simulink model "BANSHEE"  (Simulink 8.1)
settings: Solver=ode1  StartTime=0.0  StopTime=inf  FixedStep=Ts  MaxStep=1e-3  RelTol=1e-3
PostLoadFcn:
  | BANSHEE_init;
InitFcn:
  | BANSHEE_init;
undefined symbols (not defined in the file or in its folder): cable_spec, F1, F2, F3, fdesignblkfcn, Feeder1_lib, Feeder2_lib, Feeder3_lib, gcbh, generic_ethernet_cb, Left, relay_housing_lib, SM_UtilityService, SS_F1_RELAY_HOUSING, SS_F2_RELAY_HOUSING, SS_F3_RELAY_HOUSING, SS_Feeder1, SS_Feeder2, SS_Feeder3, Ts, type, utility_service_lib, V
libraries: breaker_lib x51, rtio_generic_modbus x43, relay_modbus_lib x42, cables_lib x34, artemis x24, transformer_lib x24, Load_lib x20, simulink x16, ssn_lib x16, rtlab x15, rtio_opalrt_common x15, PQFV_lib x8
(part 4 of 5)

== system BANSHEE/SM_UtilityService/HWCtrl_IOs ==
  note: When the system uses the simulated
      | Secondary Controller the digital I/O
      | should be disabled.
  note: Copyright (c) 2016 Massachusetts Institute of Technology
      | Permission is hereby granted, free of charge, to any person obtaining a copy of this software and associated documentation files (the "Software"), to deal
      | in the Software without restriction, including without limitation the rights to use, copy, modify, merge, publish, distribute, sublicense, and/or sell copies of the
      | Software, and to permit persons to whom the Software is furnished to do so, subject to the following conditions:
      |
      | THE SOFTWARE IS PROVIDED "AS IS", WITHOUT WARRANTY OF ANY KIND, EXPRESS OR IMPLIED, INCLUDING BUT NOT LIMITED TO THE
      | WARRANTIES OF MERCHANTABILITY, FITNESS FOR A PARTICULAR PURPOSE AND NONINFRINGEMENT. IN NO EVENT SHALL THE AUTHORS
      | OR COPYRIGHT HOLDERS BE LIABLE FOR ANY CLAIM, DAMAGES OR OTHER LIABILITY, WHETHER IN AN ACTION OF CONTRACT, TORT OR
      | OTHERWISE, ARISING FROM, OUT OF OR IN CONNECTION WITH THE SOFTWARE OR THE USE OR OTHER DEALINGS IN THE SOFTWARE
  ScaledSignals : Inport
  Bus Creator : BusCreator
  Bus Creator1 : BusCreator  Inputs=5
  Bus Creator2 : BusCreator  Inputs=5
  Bus Creator3 : BusCreator  Inputs=2
  Bus Selector1 : BusSelector  OutputSignals=MCB_CB_Status
  Bus Selector2 : BusSelector  OutputSignals=scaled_gcb_voltage,scaled_gcb_current,scaled_mcb_voltage,scaled_mcb_current,scaled_speed
  Bus Selector3 : BusSelector  OutputSignals=NGCHP_ScaledSignals,Diesel_ScaledSignals
  Bus Selector4 : BusSelector  OutputSignals=scaled_gcb_voltage,scaled_gcb_current,scaled_mcb_voltage,scaled_mcb_current,scaled_speed
  Bus Selector5 : BusSelector  OutputSignals=MCB_CB_Status
  Demux1 : Demux  Outputs=16
  GR1 B AIN (CH00-15) : Subsystem
  Memory1 : Memory
  OpCtrl : rtio_opalrt_common/OpCtrl  CtrlName='OpCtrl'  boardid=0  BitstreamFilename=VC707_2-EX-0001-2_3_2_20-48AIO16DIO16DIOSel-02-01.bin  numconfig=-1  mode=Master  externalClock=off  decimRtsi=0  calibIO=off  SampleTime=0  loadinport=-1  BoardType=VC707  SecondaryPresent=off  sync_type=Audio
  Woodward Inputs : Subsystem
  Woodward Outputs - Diesel - Gen2 : Subsystem
  Woodward Outputs - NGCHP - Gen1 : Subsystem
  WoodwardBias : Outport
  wires:
  Bus Creator/1 -> [WoodwardBias]
  Memory1/1 -> WoodwardBias/1
  Bus Selector1/1 -> Woodward Outputs - NGCHP - Gen1/1(Gen1 MCB Status)  "<MCB_CB_Status>"
  [NGCHP_ScaledSignals] -> Bus Selector1/1
  [WoodwardBias] -> Woodward Outputs - NGCHP - Gen1/2(WoodwardBias)
  Woodward Outputs - NGCHP - Gen1/5(Gen1 MCB) -> Bus Creator2/5  "MCB_Ctrl"
  Woodward Outputs - Diesel - Gen2/1(Digital Inputs) -> Bus Creator1/1  "DIN"
  Woodward Outputs - NGCHP - Gen1/4(Gen1 GCB) -> Bus Creator2/4  "GCB_Crtl"
  Woodward Outputs - NGCHP - Gen1/3(Gen1 Fuel Enable) -> Bus Creator2/3  "FuelEnable"
  Woodward Outputs - NGCHP - Gen1/2(Gen1 Gov and AVR) -> Bus Creator2/2  "Gov_and_AVR"
  Woodward Outputs - NGCHP - Gen1/1(Digital Inputs) -> Bus Creator2/1  "DIN"
  Bus Creator2/1 -> Bus Creator3/1  "NGCHP_Gen1"
  Bus Creator3/1 -> Memory1/1
  Bus Creator1/1 -> Bus Creator3/2  "Diesel_Gen2"
  Woodward Outputs - Diesel - Gen2/5(Gen2 MCB) -> Bus Creator1/5  "MCB_Ctrl"
  Woodward Outputs - Diesel - Gen2/4(Gen2 GCB) -> Bus Creator1/4  "GCB_Crtl"
  Woodward Outputs - Diesel - Gen2/3(Gen2 Fuel Enable) -> Bus Creator1/3  "FuelEnable"
  Woodward Outputs - Diesel - Gen2/2(Gen2 Gov and AVR) -> Bus Creator1/2  "Gov_and_AVR"
  [Diesel_ScaledSignals] -> Bus Selector5/1
  [WoodwardBias] -> Woodward Outputs - Diesel - Gen2/2(WoodwardBias)
  Bus Selector5/1 -> Woodward Outputs - Diesel - Gen2/1(Gen2 MCB Status)  "<MCB_CB_Status>"
  Demux1/4 -> Bus Creator/4  "gen2_AVR_bias"
  Demux1/3 -> Bus Creator/3  "gen2_GOV_bias"
  Demux1/2 -> Bus Creator/2  "gen1_AVR_bias"
  Demux1/1 -> Bus Creator/1  "gen1_GOV_bias"
  GR1 B AIN (CH00-15)/1(Out1) -> Demux1/1
  Bus Selector4/5 -> Woodward Inputs/10(MPU2_speed)  "<scaled_speed>"
  Bus Selector4/4 -> Woodward Inputs/9(Mains2_Current)  "<scaled_mcb_current>"
  Bus Selector4/3 -> Woodward Inputs/8(Mains2_Voltage)  "<scaled_mcb_voltage>"
  Bus Selector4/2 -> Woodward Inputs/7(Generator2_Current)  "<scaled_gcb_current>"
  Bus Selector4/1 -> Woodward Inputs/6(Generator2_Voltage)  "<scaled_gcb_voltage>"
  [Diesel_ScaledSignals] -> Bus Selector4/1
  Bus Selector2/1 -> Woodward Inputs/1(Generator1_Voltage)  "<scaled_gcb_voltage>"
  Bus Selector2/2 -> Woodward Inputs/2(Generator1_Current)  "<scaled_gcb_current>"
  Bus Selector2/3 -> Woodward Inputs/3(Mains1_Voltage)  "<scaled_mcb_voltage>"
  Bus Selector2/4 -> Woodward Inputs/4(Mains1_Current)  "<scaled_mcb_current>"
  Bus Selector2/5 -> Woodward Inputs/5(MPU1_speed)  "<scaled_speed>"
  [NGCHP_ScaledSignals] -> Bus Selector2/1
  Bus Selector3/2 -> [Diesel_ScaledSignals]  "<Diesel_ScaledSignals>"
  Bus Selector3/1 -> [NGCHP_ScaledSignals]  "<NGCHP_ScaledSignals>"
  ScaledSignals/1 -> Bus Selector3/1

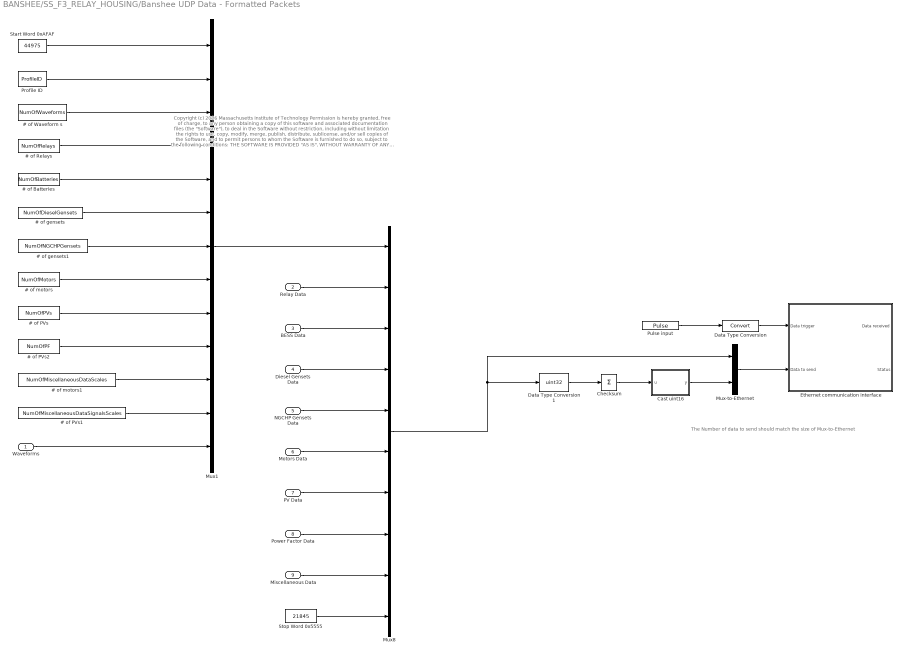
== system BANSHEE/SS_F3_RELAY_HOUSING/Banshee UDP Data - Formatted Packets ==
  note: The Number of data to send should match the size of Mux-to-Ethernet
  note: Copyright (c) 2016 Massachusetts Institute of Technology
      | Permission is hereby granted, free of charge, to any person obtaining a copy of this software and associated documentation files (the "Software"), to deal
      | in the Software without restriction, including without limitation the rights to use, copy, modify, merge, publish, distribute, sublicense, and/or sell copies of the
      | Software, and to permit persons to whom the Software is furnished to do so, subject to the following conditions:
      |
      | THE SOFTWARE IS PROVIDED "AS IS", WITHOUT WARRANTY OF ANY KIND, EXPRESS OR IMPLIED, INCLUDING BUT NOT LIMITED TO THE
      | WARRANTIES OF MERCHANTABILITY, FITNESS FOR A PARTICULAR PURPOSE AND NONINFRINGEMENT. IN NO EVENT SHALL THE AUTHORS
      | OR COPYRIGHT HOLDERS BE LIABLE FOR ANY CLAIM, DAMAGES OR OTHER LIABILITY, WHETHER IN AN ACTION OF CONTRACT, TORT OR
      | OTHERWISE, ARISING FROM, OUT OF OR IN CONNECTION WITH THE SOFTWARE OR THE USE OR OTHER DEALINGS IN THE SOFTWARE
  Waveforms : Inport  PortDimensions=3
  Relay Data : Inport  Port=2
  BESS Data : Inport  Port=3
  Diesel Gensets Data : Inport  Port=4
  NGCHP Gensets Data : Inport  Port=5
  Motors Data : Inport  Port=6
  PV Data : Inport  Port=7
  Power Factor Data : Inport  Port=8
  Miscellaneous Data : Inport  Port=9
  " # of motors" : Constant  Value=NumOfMotors  OutDataTypeStr=double
  " # of motors1" : Constant  Value=NumOfMiscellaneousDataScales  OutDataTypeStr=double
  # of Batteries : Constant  Value=NumOfBatteries  OutDataTypeStr=double
  # of PVs : Constant  Value=NumOfPVs  OutDataTypeStr=double
  # of PVs1 : Constant  Value=NumOfMiscellaneousDataSignalsScales  OutDataTypeStr=double
  # of PVs2 : Constant  Value=NumOfPF  OutDataTypeStr=double
  # of Relays : Constant  Value=NumOfRelays  OutDataTypeStr=double
  # of Waveform s : Constant  Value=NumOfWaveforms  OutDataTypeStr=double
  # of gensets : Constant  Value=NumOfDieselGensets  OutDataTypeStr=double
  # of gensets1 : Constant  Value=NumOfNGCHPGensets  OutDataTypeStr=double
  Cast uint16 : MATLAB Function  TreatAsAtomicUnit=on
  Checksum : Sum  Inputs=+
  Data Type Conversion : DataTypeConversion
  Data Type Conversion1 : DataTypeConversion  OutDataTypeStr=uint32  ConvertRealWorld=Stored Integer (SI)  RndMeth=Nearest
  Ethernet communication interface : Subsystem  mask(AsyncEthernet){ctrl_id=1, nbr_to_remote_endpoint=295, type_to_remote_endpoint=INT16, offset_to_remote_endpoint=0, swap_tx=off, nbr_from_remote_endpoint=4, type_from_remote_endpoint=UINT16, offset_from_remote_endpoint=0, swap_rx=off, exe_name='AsyncEthernet', nic_name='eth0', protocol=UDP, tcp_mode=Server, port=7200, remote_ip='255.255.255.255'}
      mask prompts: ctrl_id "Controller ID"; nbr_to_remote_endpoint "Number of data to send"; type_to_remote_endpoint "Type of data to send"; offset_to_remote_endpoint "Byte offset of transmission buffer"; swap_tx "Swap data endianness before transmission"; nbr_from_remote_endpoint "Number of data expected to be received"; type_from_remote_endpoint "Type of data expected to be received"; offset_from_remote_endpoint "Byte offset of reception buffer"; swap_rx "Swap data endianness after reception"; exe_name "Executable name"; nic_name "Network interface name"; tcp_mode "TCP mode"; port "Port number"; remote_ip "Remote IP address"
      mask help: This block is used as a communication interface to send data to a remote dedevice and receive data from it.
      mask Help: eval('rtlab_io_help(''Generic/Ethernet/Ethernet_interface.htm'');');
      mask Callback ctrl_id:
      | var = get_param(gcb,'ctrl_id');
      | set_param([gcb '/AsyncEthernetCtrl'],'ctrl_id',var)
      mask Callback nbr_to_remote_endpoint:
      | var = get_param(gcb,'nbr_to_remote_endpoint');
      | set_param([gcb '/AsyncEthernetCtrl'],'nbr_to_remote_endpoint',var)
      mask TypeOptions type_to_remote_endpoint: UINT8 | INT8 | UINT16 | INT16 | UINT32 | INT32 | FLOAT | DOUBLE
      mask Callback type_to_remote_endpoint:
      | var = get_param(gcb,'type_to_remote_endpoint');
      | set_param([gcb '/AsyncEthernetCtrl'],'type_to_remote_endpoint',var)
      mask Callback offset_to_remote_endpoint:
      | var = get_param(gcb,'offset_to_remote_endpoint');
      | set_param([gcb '/AsyncEthernetCtrl'],'offset_to_remote_endpoint',var)
      mask Callback swap_tx:
      | var = get_param(gcb,'swap_tx');
      | set_param([gcb '/AsyncEthernetCtrl'],'swap_tx',var)
      mask Callback nbr_from_remote_endpoint:
      | var = get_param(gcb,'nbr_from_remote_endpoint');
      | set_param([gcb '/AsyncEthernetCtrl'],'nbr_from_remote_endpoint',var)
      mask TypeOptions type_from_remote_endpoint: UINT8 | INT8 | UINT16 | INT16 | UINT32 | INT32 | FLOAT | DOUBLE
      mask Callback type_from_remote_endpoint:
      | var = get_param(gcb,'type_from_remote_endpoint');
      | set_param([gcb '/AsyncEthernetCtrl'],'type_from_remote_endpoint',var)
      mask Callback offset_from_remote_endpoint:
      | var = get_param(gcb,'offset_from_remote_endpoint');
      | set_param([gcb '/AsyncEthernetCtrl'],'offset_from_remote_endpoint',var)
      mask Callback swap_rx:
      | var = get_param(gcb,'swap_rx');
      | set_param([gcb '/AsyncEthernetCtrl'],'swap_rx',var)
      mask Callback exe_name:
      | str = get_param(gcb,'exe_name');
      | 
      | if exist('str','var')
      |     str = eval(str);
      | end
      | 
      | set_param([gcb '/AsyncEthernetCtrl'],'exe_name',str)
      mask Callback nic_name:
      | str = get_param(gcb,'nic_name');
      | 
      | if exist('str','var')
      |     str = eval(str);
      | end
      | 
      | set_param([gcb '/AsyncEthernetCtrl'],'nic_name',str)
      mask TypeOptions protocol: UDP | TCP
      mask Callback protocol: generic_ethernet_cb('protocol')
      mask TypeOptions tcp_mode: Client | Server
      mask Callback tcp_mode: generic_ethernet_cb('tcp_mode')
      mask Callback port:
      | var = get_param(gcb,'port');
      | set_param([gcb '/AsyncEthernetCtrl'],'port',var)
      mask Callback remote_ip:
      | str = get_param(gcb,'remote_ip');
      | 
      | if exist('str','var')
      |     str = eval(str);
      | end
      | 
      | set_param([gcb '/AsyncEthernetCtrl'],'remote_ip',str)
  Mux-to-Ethernet : Mux  Inputs=2
  Mux1 : Mux  Inputs=13
  Mux8 : Mux  Inputs=10
  Profile ID : Constant  Value=ProfileID  OutDataTypeStr=double
  Pulse input : DiscretePulseGenerator  PulseType=Time based  Period=1/5
  Start Word 0xAFAF : Constant  Value=44975  OutDataTypeStr=double
  Stop Word 0x5555 : Constant  Value=21845  OutDataTypeStr=double
  wires:
  # of Waveform s/1 -> Mux1/3
  Profile ID/1 -> Mux1/2
  Start Word 0xAFAF/1 -> Mux1/1
  Pulse input/1 -> Data Type Conversion/1
  Data Type Conversion/1 -> Ethernet communication interface/1(Data trigger)
  Mux1/1 -> Mux8/1
  Checksum/1 -> Cast uint16/1(u)
  Cast uint16/1(y) -> Mux-to-Ethernet/2
  Mux-to-Ethernet/1 -> Ethernet communication interface/2(Data to send)
  Data Type Conversion1/1 -> Checksum/1
  Waveforms/1 -> Mux1/13
  # of gensets/1 -> Mux1/6
  # of Batteries/1 -> Mux1/5
  # of Relays/1 -> Mux1/4
  BESS Data/1 -> Mux8/3
  Diesel Gensets Data/1 -> Mux8/4
  Relay Data/1 -> Mux8/2
  Mux8/1 -> Mux-to-Ethernet/1, Data Type Conversion1/1
  # of gensets1/1 -> Mux1/7
  " # of motors"/1 -> Mux1/8
  # of PVs/1 -> Mux1/9
  # of PVs2/1 -> Mux1/10
  " # of motors1"/1 -> Mux1/11
  # of PVs1/1 -> Mux1/12
  Stop Word 0x5555/1 -> Mux8/10
  NGCHP Gensets Data/1 -> Mux8/5
  Miscellaneous Data/1 -> Mux8/9
  Power Factor Data/1 -> Mux8/8
  PV Data/1 -> Mux8/7
  Motors Data/1 -> Mux8/6

== system BANSHEE/SS_F3_RELAY_HOUSING/SEL751-UDP ==
  note: Order of signals:
      | F3_PCC
      | F2_PCC
      | F1_PCC
      | F3_GCB (NG/CHP)
      | F1_GCB (DIESEL)
  note: % Copyright (c) 2016 Massachusetts Institute of Technology
      | % Permission is hereby granted, free of charge, to any person obtaining a copy of this
      | % software and associated documentation files (the "Software"), to deal in the Software
      | % without restriction, including without limitation the rights to use, copy, modify,
      | % merge, publish, distribute, sublicense, and/or sell copies of the Software, and to
      | % permit persons to whom the Software is furnished to do so, subject to the following
      | % conditions:
      | %
      | %
      | % The above copyright notice and this permission notice shall be included in
      | % all copies or substantial portions of the Software.
      | %
      | % THE SOFTWARE IS PROVIDED "AS IS", WITHOUT WARRANTY OF ANY KIND, EXPRESS OR IMPLIED,
      | % INCLUDING BUT NOT LIMITED TO THE WARRANTIES OF MERCHANTABILITY, FITNESS FOR A
      | % PARTICULAR PURPOSE AND NONINFRINGEMENT. IN NO EVENT SHALL THE AUTHORS OR COPYRIGHT
      | % HOLDERS BE LIABLE FOR ANY CLAIM, DAMAGES OR OTHER LIABILITY, WHETHER IN AN ACTION
      | % OF CONTRACT, TORT OR OTHERWISE, ARISING FROM, OUT OF OR IN CONNECTION WITH THE
      | % SOFTWARE OR THE USE OR OTHER DEALINGS IN THE SOFTWARE.
      | %
      | %
      | %%
  F3_MS : Inport
  F2_MS : Inport  Port=2
  F1_MS : Inport  Port=3
  Bus Creator : BusCreator  Inputs=5
  Bus Selector : BusSelector  OutputSignals=CB_DATA.F3_PCC
  Bus Selector3 : BusSelector  OutputSignals=CB_DATA.F2_PCC
  Bus Selector5 : BusSelector  OutputSignals=CB_DATA.F1_PCC
  PQFV : PQFV_lib/PQFV  VRMSLL=13800
  PQFV1 : PQFV_lib/PQFV  VRMSLL=13800
  PQFV2 : PQFV_lib/PQFV  VRMSLL=13800
  PQVF_out : Outport
  wires:
  Bus Selector/1 -> PQFV/1  "<F3_PCC>"
  Bus Selector3/1 -> PQFV1/1  "<F2_PCC>"
  F2_MS/1 -> Bus Selector3/1
  Bus Selector5/1 -> PQFV2/1  "<F1_PCC>"
  PQFV1/1 -> Bus Creator/2  "F2_PCC"
  PQFV/1 -> Bus Creator/1  "F3_PCC"
  PQFV2/1 -> Bus Creator/3  "F1_PCC"
  F3_MS/1 -> Bus Creator/4, Bus Selector/1  "F3_MS"
  F1_MS/1 -> Bus Creator/5, Bus Selector5/1  "F1_MS"
  Bus Creator/1 -> PQVF_out/1

== system BANSHEE/SS_Feeder3/HWController_3.5MVA_NGCHP ==
  note: Copyright (c) 2016 Massachusetts Institute of Technology
      | Permission is hereby granted, free of charge, to any person obtaining a copy of this software and associated documentation files (the "Software"), to deal
      | in the Software without restriction, including without limitation the rights to use, copy, modify, merge, publish, distribute, sublicense, and/or sell copies of the
      | Software, and to permit persons to whom the Software is furnished to do so, subject to the following conditions:
      |
      | THE SOFTWARE IS PROVIDED "AS IS", WITHOUT WARRANTY OF ANY KIND, EXPRESS OR IMPLIED, INCLUDING BUT NOT LIMITED TO THE
      | WARRANTIES OF MERCHANTABILITY, FITNESS FOR A PARTICULAR PURPOSE AND NONINFRINGEMENT. IN NO EVENT SHALL THE AUTHORS
      | OR COPYRIGHT HOLDERS BE LIABLE FOR ANY CLAIM, DAMAGES OR OTHER LIABILITY, WHETHER IN AN ACTION OF CONTRACT, TORT OR
      | OTHERWISE, ARISING FROM, OUT OF OR IN CONNECTION WITH THE SOFTWARE OR THE USE OR OTHER DEALINGS IN THE SOFTWARE
  In1 : Inport
  In2 : Inport  Port=2
  HWControllerBias : Inport  Port=3
  Bus Creator2 : BusCreator  Inputs=6
  Bus Selector6 : BusSelector  OutputSignals=Heat Recovered; MBtu/hr
  Bus Selector7 : BusSelector  OutputSignals=TempActual,HeatFromBoiler MBtu/hr,CHPHeatContribution MBtu/hr,Thermal data.Heat Recovered; MBtu/hr,Thermal data.CO2 lbm/hr
  CHPThermalModel : CHP_Model_lib/CHPThermalModel  SIM_HIL=SIM_HIL
  Demux : Demux  Outputs=2
  HWController_NG_Generator : HWController_NGCHP_Genset_3p5MVA_lib/HWController_NG_Generator
  Modbus device : rtio_generic_modbus/Modbus device  conf_name=CHP_slave_cfg.opal  conf_name_mask=CHP_slave_cfg.xls  sample_time=Ts
  Mux1 : Mux  Inputs=5
  A : PMIOPort  Tag=A  Port=1  Side=Right
      settings: AttributesFormatString=A
  B : PMIOPort  Port=2  Side=Right
  C : PMIOPort  Port=3  Side=Right
  Out1 : Outport
  Generator Data : Outport  Port=2
  GCB Control : Outport  Port=3
  wires:
  In2/1 -> CHPThermalModel/5  "CHP_SIM_Cmds"
  Bus Creator2/1 -> Bus Selector7/1, Out1/1  "CHPData"
  Bus Selector6/1 -> CHPThermalModel/1  "<Heat Recovered; MBtu/hr>"
  HWController_NG_Generator/2 -> GCB Control/1
  HWController_NG_Generator/1 -> Generator Data/1
  Modbus device/2 -> Demux/1
  [HeatRec_MBtuhr] -> Bus Selector6/1, Bus Creator2/2  "Thermal data"
  CHPThermalModel/3 -> Bus Creator2/4
  Demux/1 -> CHPThermalModel/3
  Mux1/1 -> Modbus device/4
  In1/1 -> CHPThermalModel/2
  Bus Selector7/1 -> Mux1/1  "<TempActual>"
  Bus Selector7/4 -> Mux1/4  "<Heat Recovered; MBtu/hr>"
  Bus Selector7/5 -> Mux1/5  "<CO2 lbm/hr>"
  Bus Selector7/2 -> Mux1/2  "<HeatFromBoiler MBtu/hr>"
  CHPThermalModel/2 -> Bus Creator2/3
  Demux/2 -> CHPThermalModel/4
  CHPThermalModel/1 -> Bus Creator2/1  "TempActual"
  Bus Selector7/3 -> Mux1/3  "<CHPHeatContribution MBtu/hr>"
  HWController_NG_Generator/3 -> [HeatRec_MBtuhr]  "Thermal data"
  HWControllerBias/1 -> HWController_NG_Generator/1
  CHPThermalModel/4 -> Bus Creator2/5
  CHPThermalModel/5 -> Bus Creator2/6
  connections:
  HWController_NG_Generator/RConn1 -- A/RConn1
  HWController_NG_Generator/RConn2 -- B/RConn1
  HWController_NG_Generator/RConn3 -- C/RConn1

== system BANSHEE/SC_ctrl/Overall/currents ==
  F1 : Inport
  F2 : Inport  Port=2
  F3 : Inport  Port=3
  1ph_rms1 : Subsystem
  1ph_rms10 : Subsystem
  1ph_rms11 : Subsystem
  1ph_rms12 : Subsystem
  1ph_rms13 : Subsystem
  1ph_rms14 : Subsystem
  1ph_rms15 : Subsystem
  1ph_rms2 : Subsystem
  1ph_rms3 : Subsystem
  1ph_rms4 : Subsystem
  1ph_rms5 : Subsystem
  1ph_rms6 : Subsystem
  1ph_rms7 : Subsystem
  1ph_rms8 : Subsystem
  1ph_rms9 : Subsystem
  Bus Selector : BusSelector  OutputSignals=F1_CB_1.m.Iabc,F1_CB_2.m.Iabc,F1_CB_3.m.Iabc,F1_CB_6.m.Iabc,F1_CB_10.m.Iabc
  Bus Selector1 : BusSelector  OutputSignals=F2_CB_1.m.Iabc,F2_CB_2.m.Iabc,F2_CB_3.m.Iabc,F2_CB_7.m.Iabc,F2_CB_14.m.Iabc,F2_CB_15.m.Iabc
  Bus Selector2 : BusSelector  OutputSignals=F3_CB_1.m.Iabc,F3_CB_2.m.Iabc,F3_CB_3.m.Iabc,F3_CB_4.m.Iabc
  Mux : Mux  Inputs=5
  Mux1 : Mux  Inputs=6
  Mux2 : Mux
  RMS_Calculator : Subsystem
  RMS_Calculator1 : Subsystem
  RMS_Calculator2 : Subsystem
  oF1 : Outport
  oF2 : Outport  Port=2
  oF3 : Outport  Port=3
  wires:
  Mux/1 -> RMS_Calculator/1(Signal)  "F1"
  Mux1/1 -> RMS_Calculator1/1(Signal)  "F2"
  Mux2/1 -> RMS_Calculator2/1(Signal)  "F3"
  Bus Selector/5 -> 1ph_rms3/1(i)  "<Iabc>"
  Bus Selector/4 -> 1ph_rms4/1(i)  "<Iabc>"
  Bus Selector/3 -> 1ph_rms2/1(i)  "<Iabc>"
  Bus Selector/2 -> 1ph_rms1/1(i)  "<Iabc>"
  Bus Selector/1 -> 1ph_rms6/1(i)  "<Iabc>"
  Bus Selector1/4 -> 1ph_rms9/1(i)  "<Iabc>"
  Bus Selector1/5 -> 1ph_rms13/1(i)  "<Iabc>"
  Bus Selector1/3 -> 1ph_rms8/1(i)  "<Iabc>"
  Bus Selector1/6 -> 1ph_rms10/1(i)  "<Iabc>"
  Bus Selector1/2 -> 1ph_rms7/1(i)  "<Iabc>"
  Bus Selector1/1 -> 1ph_rms5/1(i)  "<Iabc>"
  Bus Selector2/4 -> 1ph_rms15/1(i)  "<Iabc>"
  Bus Selector2/2 -> 1ph_rms12/1(i)  "<Iabc>"
  Bus Selector2/3 -> 1ph_rms11/1(i)  "<Iabc>"
  Bus Selector2/1 -> 1ph_rms14/1(i)  "<Iabc>"
  1ph_rms6/1(o) -> Mux/1
  1ph_rms1/1(o) -> Mux/2
  1ph_rms2/1(o) -> Mux/3
  1ph_rms3/1(o) -> Mux/5
  1ph_rms4/1(o) -> Mux/4
  1ph_rms5/1(o) -> Mux1/1
  1ph_rms7/1(o) -> Mux1/2
  1ph_rms8/1(o) -> Mux1/3
  1ph_rms9/1(o) -> Mux1/4
  1ph_rms14/1(o) -> Mux2/1
  1ph_rms13/1(o) -> Mux1/5
  1ph_rms10/1(o) -> Mux1/6
  1ph_rms12/1(o) -> Mux2/2
  1ph_rms11/1(o) -> Mux2/3
  1ph_rms15/1(o) -> Mux2/4
  RMS_Calculator/1(RMS_Signal) -> oF1/1
  RMS_Calculator1/1(RMS_Signal) -> oF2/1
  RMS_Calculator2/1(RMS_Signal) -> oF3/1
  F1/1 -> Bus Selector/1
  F2/1 -> Bus Selector1/1
  F3/1 -> Bus Selector2/1

== system BANSHEE/SC_ctrl/Overall/voltages ==
  F1 : Inport
  F2 : Inport  Port=2
  F3 : Inport  Port=3
  Bus Selector : BusSelector  OutputSignals=F1_CB_1.m.Vpu,F1_CB_2.m.Vpu,F1_CB_3.m.Vpu,F1_CB_4.m.Vpu,F1_CB_5.m.Vpu,F1_CB_6.m.Vpu,F1_CB_7.m.Vpu,F1_CB_8.m.Vpu,F1_CB_9.m.Vpu,F1_CB_10.m.Vpu,F1_CB_11.m.Vpu,F1_CB_12.m.Vpu,F1_CB_13.m.Vpu,F1_CB_14.m.Vpu
  Bus Selector1 : BusSelector  OutputSignals=F2_CB_1.m.Vpu,F2_CB_2.m.Vpu,F2_CB_3.m.Vpu,F2_CB_4.m.Vpu,F2_CB_5.m.Vpu,F2_CB_6.m.Vpu,F2_CB_7.m.Vpu,F2_CB_8.m.Vpu,F2_CB_9.m.Vpu,F2_CB_10.m.Vpu,F2_CB_11.m.Vpu,F2_CB_12.m.Vpu,F2_CB_13.m.Vpu,F2_CB_14.m.Vpu,F2_CB_15.m.Vpu,F2_CB_16.m.Vpu,F2_CB_17.m.Vpu,F2_CB_18.m.Vpu,F2_CB_19.m.Vpu
  Bus Selector2 : BusSelector  OutputSignals=F3_CB_1.m.Vpu,F3_CB_2.m.Vpu,F3_CB_3.m.Vpu,F3_CB_4.m.Vpu,F3_CB_5.m.Vpu,F3_CB_6.m.Vpu,F3_CB_7.m.Vpu,F3_CB_8.m.Vpu,F3_CB_9.m.Vpu
  Mux : Mux  Inputs=14
  Mux1 : Mux  Inputs=19
  Mux2 : Mux  Inputs=9
  oF1 : Outport
  oF2 : Outport  Port=2
  oF3 : Outport  Port=3
  wires:
  Mux/1 -> oF1/1  "F1"
  F1/1 -> Bus Selector/1
  Mux1/1 -> oF2/1  "F2"
  F2/1 -> Bus Selector1/1
  Mux2/1 -> oF3/1  "F3"
  F3/1 -> Bus Selector2/1
  Bus Selector/14 -> Mux/14  "<Vpu>"
  Bus Selector/6 -> Mux/6  "<Vpu>"
  Bus Selector/5 -> Mux/5  "<Vpu>"
  Bus Selector/10 -> Mux/10  "<Vpu>"
  Bus Selector/4 -> Mux/4  "<Vpu>"
  Bus Selector/9 -> Mux/9  "<Vpu>"
  Bus Selector/7 -> Mux/7  "<Vpu>"
  Bus Selector/2 -> Mux/2  "<Vpu>"
  Bus Selector/1 -> Mux/1  "<Vpu>"
  Bus Selector/3 -> Mux/3  "<Vpu>"
  Bus Selector/13 -> Mux/13  "<Vpu>"
  Bus Selector/12 -> Mux/12  "<Vpu>"
  Bus Selector/11 -> Mux/11  "<Vpu>"
  Bus Selector/8 -> Mux/8  "<Vpu>"
  Bus Selector1/19 -> Mux1/19  "<Vpu>"
  Bus Selector1/18 -> Mux1/18  "<Vpu>"
  Bus Selector1/7 -> Mux1/7  "<Vpu>"
  Bus Selector1/10 -> Mux1/10  "<Vpu>"
  Bus Selector1/11 -> Mux1/11  "<Vpu>"
  Bus Selector1/2 -> Mux1/2  "<Vpu>"
  Bus Selector1/13 -> Mux1/13  "<Vpu>"
  Bus Selector1/14 -> Mux1/14  "<Vpu>"
  Bus Selector1/15 -> Mux1/15  "<Vpu>"
  Bus Selector1/6 -> Mux1/6  "<Vpu>"
  Bus Selector1/4 -> Mux1/4  "<Vpu>"
  Bus Selector1/3 -> Mux1/3  "<Vpu>"
  Bus Selector1/1 -> Mux1/1  "<Vpu>"
  Bus Selector1/5 -> Mux1/5  "<Vpu>"
  Bus Selector1/8 -> Mux1/8  "<Vpu>"
  Bus Selector1/12 -> Mux1/12  "<Vpu>"
  Bus Selector1/16 -> Mux1/16  "<Vpu>"
  Bus Selector1/17 -> Mux1/17  "<Vpu>"
  Bus Selector1/9 -> Mux1/9  "<Vpu>"
  Bus Selector2/5 -> Mux2/5  "<Vpu>"
  Bus Selector2/4 -> Mux2/4  "<Vpu>"
  Bus Selector2/6 -> Mux2/6  "<Vpu>"
  Bus Selector2/3 -> Mux2/3  "<Vpu>"
  Bus Selector2/7 -> Mux2/7  "<Vpu>"
  Bus Selector2/8 -> Mux2/8  "<Vpu>"
  Bus Selector2/2 -> Mux2/2  "<Vpu>"
  Bus Selector2/9 -> Mux2/9  "<Vpu>"
  Bus Selector2/1 -> Mux2/1  "<Vpu>"

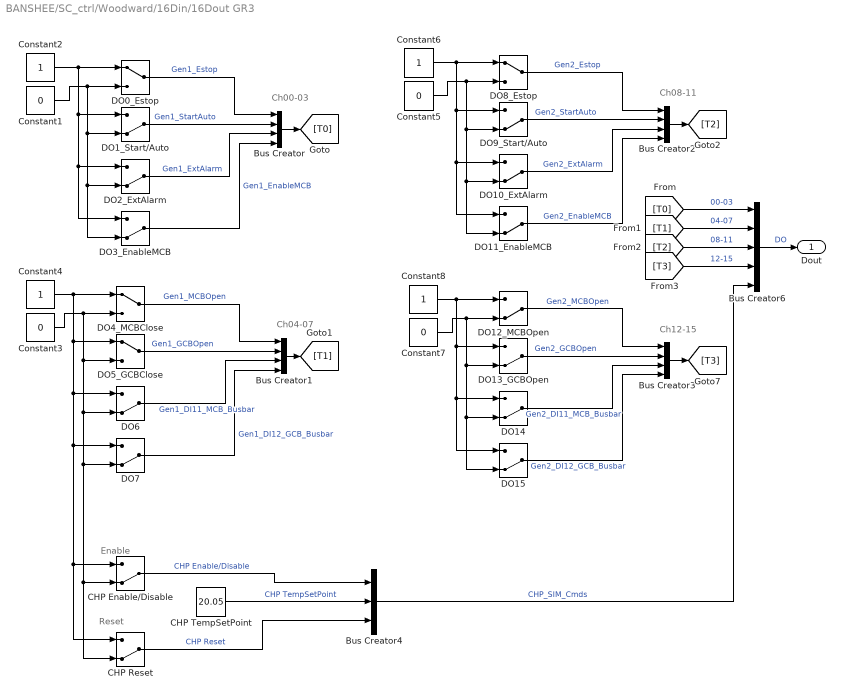
== system BANSHEE/SC_ctrl/Woodward/16Din/16Dout GR3 ==
  note: Ch00-03
  note: Ch04-07
  note: Ch08-11
  note: Ch12-15
  note: Enable
  note: Reset
  Bus Creator{,1..3} (4 alike) : BusCreator
  Bus Creator4 : BusCreator  Inputs=3
  Bus Creator6 : BusCreator  Inputs=5
  CHP Enable/Disable : ManualSwitch  CurrentSetting=0
  CHP Reset : ManualSwitch  CurrentSetting=0
  CHP TempSetPoint : Constant  Value=20.05
  Constant{1,3,5,7} (4 alike) : Constant  Value=0
  Constant{2,4,6,8} (4 alike) : Constant
  DO0_Estop : ManualSwitch
  DO10_ExtAlarm : ManualSwitch  CurrentSetting=0
  DO11_EnableMCB : ManualSwitch  CurrentSetting=0
  DO12_MCBOpen : ManualSwitch  CurrentSetting=0
  DO13_GCBOpen : ManualSwitch  CurrentSetting=0
  DO{6..7,14..15} (4 alike) : ManualSwitch  CurrentSetting=0
  DO1_Start/Auto : ManualSwitch  CurrentSetting=0
  DO2_ExtAlarm : ManualSwitch  CurrentSetting=0
  DO3_EnableMCB : ManualSwitch  CurrentSetting=0
  DO4_MCBClose : ManualSwitch
  DO5_GCBClose : ManualSwitch
  DO8_Estop : ManualSwitch
  DO9_Start/Auto : ManualSwitch  CurrentSetting=0
  Dout : Outport
  wires:
  Bus Creator4/1 -> Bus Creator6/5  "CHP_SIM_Cmds"
  CHP Reset/1 -> Bus Creator4/3  "CHP Reset"
  CHP TempSetPoint/1 -> Bus Creator4/2  "CHP TempSetPoint"
  CHP Enable/Disable/1 -> Bus Creator4/1  "CHP Enable/Disable"
  Bus Creator6/1 -> Dout/1  "DO"
  Constant2/1 -> DO0_Estop/1, DO1_Start/Auto/1, DO3_EnableMCB/1, DO2_ExtAlarm/1
  Constant1/1 -> DO0_Estop/2, DO1_Start/Auto/2, DO3_EnableMCB/2, DO2_ExtAlarm/2
  DO0_Estop/1 -> Bus Creator/1  "Gen1_Estop"
  DO1_Start/Auto/1 -> Bus Creator/2  "Gen1_StartAuto"
  DO2_ExtAlarm/1 -> Bus Creator/3  "Gen1_ExtAlarm"
  DO3_EnableMCB/1 -> Bus Creator/4  "Gen1_EnableMCB"
  Constant4/1 -> DO6/1, DO7/1, CHP Enable/Disable/1, CHP Reset/1, DO5_GCBClose/1, DO4_MCBClose/1
  Constant3/1 -> DO6/2, CHP Enable/Disable/2, CHP Reset/2, DO7/2, DO5_GCBClose/2, DO4_MCBClose/2
  DO4_MCBClose/1 -> Bus Creator1/1  "Gen1_MCBOpen"
  DO5_GCBClose/1 -> Bus Creator1/2  "Gen1_GCBOpen"
  DO6/1 -> Bus Creator1/3  "Gen1_DI11_MCB_Busbar"
  DO7/1 -> Bus Creator1/4  "Gen1_DI12_GCB_Busbar"
  Constant6/1 -> DO8_Estop/1, DO9_Start/Auto/1, DO11_EnableMCB/1, DO10_ExtAlarm/1
  Constant5/1 -> DO8_Estop/2, DO9_Start/Auto/2, DO11_EnableMCB/2, DO10_ExtAlarm/2
  DO8_Estop/1 -> Bus Creator2/1  "Gen2_Estop"
  DO9_Start/Auto/1 -> Bus Creator2/2  "Gen2_StartAuto"
  DO10_ExtAlarm/1 -> Bus Creator2/3  "Gen2_ExtAlarm"
  DO11_EnableMCB/1 -> Bus Creator2/4  "Gen2_EnableMCB"
  Constant8/1 -> DO14/1, DO15/1, DO13_GCBOpen/1, DO12_MCBOpen/1
  Constant7/1 -> DO14/2, DO15/2, DO13_GCBOpen/2, DO12_MCBOpen/2
  DO12_MCBOpen/1 -> Bus Creator3/1  "Gen2_MCBOpen"
  DO13_GCBOpen/1 -> Bus Creator3/2  "Gen2_GCBOpen"
  DO14/1 -> Bus Creator3/3  "Gen2_DI11_MCB_Busbar"
  DO15/1 -> Bus Creator3/4  "Gen2_DI12_GCB_Busbar"
  Bus Creator/1 -> [T0]
  Bus Creator1/1 -> [T1]
  Bus Creator3/1 -> [T3]
  Bus Creator2/1 -> [T2]
  [T0] -> Bus Creator6/1  "00-03"
  [T1] -> Bus Creator6/2  "04-07"
  [T2] -> Bus Creator6/3  "08-11"
  [T3] -> Bus Creator6/4  "12-15"

== system BANSHEE/SM_UtilityService/HWCtrl_IOs/GR1 B AIN (CH00-15) ==
  AnalogIn : rtio_opalrt_common/AnalogIn  CtrlName='OpCtrl'  portNb=1  FcnNos=Slot 1 Module B Subsection 1  size=16  maxcount=8  count=8  numchan=8  sampleTime=0
      settings: AttributesFormatString=%<CtrlName>
  AnalogIn1 : rtio_opalrt_common/AnalogIn  CtrlName='OpCtrl'  portNb=2  FcnNos=Slot 1 Module B Subsection 2  size=16  maxcount=8  count=8  numchan=8  sampleTime=0
      settings: AttributesFormatString=%<CtrlName>
  Mux6 : Mux  Inputs=2
  Terminator2 : Terminator
  Terminator3 : Terminator
  Out1 : Outport
  wires:
  Mux6/1 -> Out1/1
  AnalogIn1/2 -> Terminator3/1
  AnalogIn/2 -> Terminator2/1
  AnalogIn1/1 -> Mux6/2
  AnalogIn/1 -> Mux6/1

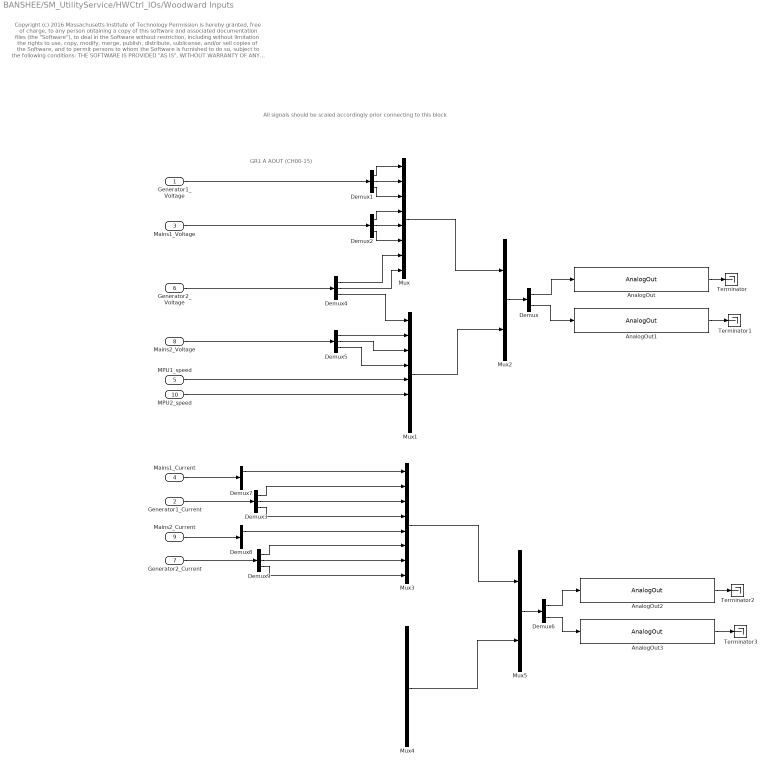
== system BANSHEE/SM_UtilityService/HWCtrl_IOs/Woodward Inputs ==
  note: Copyright (c) 2016 Massachusetts Institute of Technology
      | Permission is hereby granted, free of charge, to any person obtaining a copy of this software and associated documentation files (the "Software"), to deal
      | in the Software without restriction, including without limitation the rights to use, copy, modify, merge, publish, distribute, sublicense, and/or sell copies of the
      | Software, and to permit persons to whom the Software is furnished to do so, subject to the following conditions:
      |
      | THE SOFTWARE IS PROVIDED "AS IS", WITHOUT WARRANTY OF ANY KIND, EXPRESS OR IMPLIED, INCLUDING BUT NOT LIMITED TO THE
      | WARRANTIES OF MERCHANTABILITY, FITNESS FOR A PARTICULAR PURPOSE AND NONINFRINGEMENT. IN NO EVENT SHALL THE AUTHORS
      | OR COPYRIGHT HOLDERS BE LIABLE FOR ANY CLAIM, DAMAGES OR OTHER LIABILITY, WHETHER IN AN ACTION OF CONTRACT, TORT OR
      | OTHERWISE, ARISING FROM, OUT OF OR IN CONNECTION WITH THE SOFTWARE OR THE USE OR OTHER DEALINGS IN THE SOFTWARE
  note: GR1 A AOUT (CH00-15)
  note: All signals should be scaled accordingly prior connecting to this block
  Generator1_Voltage : Inport
  Generator1_Current : Inport  Port=2
  Mains1_Voltage : Inport  Port=3
  Mains1_Current : Inport  Port=4
  MPU1_speed : Inport  Port=5
  Generator2_Voltage : Inport  Port=6
  Generator2_Current : Inport  Port=7
  Mains2_Voltage : Inport  Port=8
  Mains2_Current : Inport  Port=9
  MPU2_speed : Inport  Port=10
  AnalogOut : rtio_opalrt_common/AnalogOut  CtrlName='OpCtrl'  portNb=1  FcnNos=Slot 1 Module A Subsection 1  size=16  maxcount=8  count=8  numchan=8  israngeinput=off  voltagerange=[-16 ... 16]  slot=0  side=0  mismatch=0  slotside=Slot_1_Module_A
      settings: AttributesFormatString=%<CtrlName>
  AnalogOut1 : rtio_opalrt_common/AnalogOut  CtrlName='OpCtrl'  portNb=2  FcnNos=Slot 1 Module A Subsection 2  size=16  maxcount=8  count=8  numchan=8  israngeinput=off  voltagerange=[-16 ... 16]  slot=0  side=0  mismatch=0  slotside=Slot_1_Module_A
      settings: AttributesFormatString=%<CtrlName>
  AnalogOut2 : rtio_opalrt_common/AnalogOut  CtrlName='OpCtrl'  portNb=3  FcnNos=Slot 2 Module A Subsection 1  size=16  maxcount=8  count=8  numchan=8  israngeinput=off  voltagerange=[-16 ... 16]  slot=1  side=0  mismatch=0  slotside=Slot_2_Module_A
      settings: AttributesFormatString=%<CtrlName>
  AnalogOut3 : rtio_opalrt_common/AnalogOut  CtrlName='OpCtrl'  portNb=4  FcnNos=Slot 2 Module A Subsection 2  size=16  maxcount=8  count=8  numchan=8  israngeinput=off  voltagerange=[-16 ... 16]  slot=1  side=0  mismatch=0  slotside=Slot_2_Module_A
      settings: AttributesFormatString=%<CtrlName>
  Demux : Demux  Outputs=2
  Demux{1..5,7..9} (8 alike) : Demux  Outputs=3
  Demux6 : Demux  Outputs=2
  Mux{,1,3..4} (4 alike) : Mux  Inputs=8
  Mux2 : Mux  Inputs=2
  Mux5 : Mux  Inputs=2
  Terminator{,1..3} (4 alike) : Terminator
  wires:
  Mains1_Voltage/1 -> Demux2/1
  Generator1_Voltage/1 -> Demux1/1
  Mux2/1 -> Demux/1
  Mux1/1 -> Mux2/2
  Mux/1 -> Mux2/1
  Demux/2 -> AnalogOut1/1
  Demux/1 -> AnalogOut/1
  AnalogOut1/1 -> Terminator1/1
  AnalogOut/1 -> Terminator/1
  Demux1/1 -> Mux/1
  Demux1/2 -> Mux/2
  Demux1/3 -> Mux/3
  Demux2/1 -> Mux/4
  Demux2/2 -> Mux/5
  Demux2/3 -> Mux/6
  MPU1_speed/1 -> Mux1/5
  Demux4/1 -> Mux/7
  Demux4/2 -> Mux/8
  Demux4/3 -> Mux1/1
  Demux5/1 -> Mux1/2
  Demux5/2 -> Mux1/3
  Demux5/3 -> Mux1/4
  Mux5/1 -> Demux6/1
  Mux4/1 -> Mux5/2
  Mux3/1 -> Mux5/1
  Demux6/2 -> AnalogOut3/1
  Demux6/1 -> AnalogOut2/1
  AnalogOut3/1 -> Terminator3/1
  AnalogOut2/1 -> Terminator2/1
  Generator1_Current/1 -> Demux3/1
  Demux3/1 -> Mux3/2
  Demux3/2 -> Mux3/3
  Demux3/3 -> Mux3/4
  Mains1_Current/1 -> Demux7/1
  Demux7/1 -> Mux3/1
  Mains2_Voltage/1 -> Demux5/1
  Generator2_Voltage/1 -> Demux4/1
  MPU2_speed/1 -> Mux1/6
  Mains2_Current/1 -> Demux8/1
  Demux8/1 -> Mux3/5
  Generator2_Current/1 -> Demux9/1
  Demux9/1 -> Mux3/6
  Demux9/2 -> Mux3/7
  Demux9/3 -> Mux3/8

== system BANSHEE/SM_UtilityService/HWCtrl_IOs/Woodward Outputs - Diesel - Gen2 ==
  note: Copyright (c) 2016 Massachusetts Institute of Technology
      | Permission is hereby granted, free of charge, to any person obtaining a copy of this software and associated documentation files (the "Software"), to deal
      | in the Software without restriction, including without limitation the rights to use, copy, modify, merge, publish, distribute, sublicense, and/or sell copies of the
      | Software, and to permit persons to whom the Software is furnished to do so, subject to the following conditions:
      |
      | THE SOFTWARE IS PROVIDED "AS IS", WITHOUT WARRANTY OF ANY KIND, EXPRESS OR IMPLIED, INCLUDING BUT NOT LIMITED TO THE
      | WARRANTIES OF MERCHANTABILITY, FITNESS FOR A PARTICULAR PURPOSE AND NONINFRINGEMENT. IN NO EVENT SHALL THE AUTHORS
      | OR COPYRIGHT HOLDERS BE LIABLE FOR ANY CLAIM, DAMAGES OR OTHER LIABILITY, WHETHER IN AN ACTION OF CONTRACT, TORT OR
      | OTHERWISE, ARISING FROM, OUT OF OR IN CONNECTION WITH THE SOFTWARE OR THE USE OR OTHER DEALINGS IN THE SOFTWARE
  Gen2 MCB Status : Inport
  WoodwardBias : Inport  Port=2
  Bus Creator1 : BusCreator  Inputs=1
  DIO - Gr3 : Subsystem
  DIO - Woodward : Subsystem
  DOUT type config : Subsystem
  Woodward Primary Inputs - Gen2 : Subsystem
  Digital Inputs : Outport
  Gen2 Gov and AVR : Outport  Port=2
  Gen2 Fuel Enable : Outport  Port=3
  Gen2 GCB : Outport  Port=4
  Gen2 MCB : Outport  Port=5
  wires:
  Bus Creator1/1 -> Digital Inputs/1
  DIO - Woodward/1(DIn1) -> DIO - Gr3/1(Dout)
  DIO - Gr3/1(DIn) -> Bus Creator1/1, DIO - Woodward/1(Din_Wood)  "DIN"
  Woodward Primary Inputs - Gen2/1(Gen2 Gov and AVR) -> Gen2 Gov and AVR/1
  DIO - Woodward/3(Gen2 GCB) -> Gen2 GCB/1
  DIO - Woodward/2(Gen2 Fuel Enable) -> Gen2 Fuel Enable/1
  DIO - Woodward/4(Gen2 MCB) -> Gen2 MCB/1
  Gen2 MCB Status/1 -> DIO - Woodward/2(Gen2 MCB Status)
  WoodwardBias/1 -> Woodward Primary Inputs - Gen2/1(WoodwardBias)

== system BANSHEE/SM_UtilityService/HWCtrl_IOs/Woodward Outputs - NGCHP - Gen1 ==
  note: Copyright (c) 2016 Massachusetts Institute of Technology
      | Permission is hereby granted, free of charge, to any person obtaining a copy of this software and associated documentation files (the "Software"), to deal
      | in the Software without restriction, including without limitation the rights to use, copy, modify, merge, publish, distribute, sublicense, and/or sell copies of the
      | Software, and to permit persons to whom the Software is furnished to do so, subject to the following conditions:
      |
      | THE SOFTWARE IS PROVIDED "AS IS", WITHOUT WARRANTY OF ANY KIND, EXPRESS OR IMPLIED, INCLUDING BUT NOT LIMITED TO THE
      | WARRANTIES OF MERCHANTABILITY, FITNESS FOR A PARTICULAR PURPOSE AND NONINFRINGEMENT. IN NO EVENT SHALL THE AUTHORS
      | OR COPYRIGHT HOLDERS BE LIABLE FOR ANY CLAIM, DAMAGES OR OTHER LIABILITY, WHETHER IN AN ACTION OF CONTRACT, TORT OR
      | OTHERWISE, ARISING FROM, OUT OF OR IN CONNECTION WITH THE SOFTWARE OR THE USE OR OTHER DEALINGS IN THE SOFTWARE
  Gen1 MCB Status : Inport
  WoodwardBias : Inport  Port=2
  Bus Creator1 : BusCreator  Inputs=1
  DIO - Gr3 : Subsystem
  DIO - Woodward : Subsystem
  DOUT type config : Subsystem
  Woodward Primary Inputs - Gen1 : Subsystem
  Digital Inputs : Outport
  Gen1 Gov and AVR : Outport  Port=2
  Gen1 Fuel Enable : Outport  Port=3
  Gen1 GCB : Outport  Port=4
  Gen1 MCB : Outport  Port=5
  wires:
  DIO - Woodward/4(DIn1) -> DIO - Gr3/1(Dout)
  DIO - Gr3/1(DIn) -> DIO - Woodward/1(Din_Wood), Bus Creator1/1  "DIN"
  Bus Creator1/1 -> Digital Inputs/1
  Woodward Primary Inputs - Gen1/1(Gen1 Gov and AVR) -> Gen1 Gov and AVR/1
  WoodwardBias/1 -> Woodward Primary Inputs - Gen1/1(WoodwardBias)
  DIO - Woodward/2(Gen1 GCB) -> Gen1 GCB/1
  DIO - Woodward/3(Gen1 MCB) -> Gen1 MCB/1
  DIO - Woodward/1(Gen1 Fuel Enable) -> Gen1 Fuel Enable/1
  Gen1 MCB Status/1 -> DIO - Woodward/2(Gen1 MCB Status)

== system BANSHEE/SS_F3_RELAY_HOUSING/Banshee UDP Data - Formatted Packets/Ethernet communication interface ==
  note: Ethernet communication interface example model
  Data trigger : Inport
  Data to send : Inport  Port=2
  AsyncEthernetCtrl : S-Function  InitFcn=generic_ethernet_cb('initfcn');  FunctionName=sfun_gen_async_ctrl  Parameters=ctrl_id, nbr_to_remote_endpoint, type_to_remote_endpoint,nbr_from_remote_endpoint,type_from_remote_endpoint,protocol,tcp_mode, port, offset_to_remote_endpoint,offset_from_remote_endpoint,swap_tx,swap_rx,0,nic_name,remote_ip,'','','','','','','','','','',exe_name,0  EnableBusSupport=off  mask(AsyncEthernetCtrl){ctrl_id=1, nbr_to_remote_endpoint=295, type_to_remote_endpoint=INT16, offset_to_remote_endpoint=0, nbr_from_remote_endpoint=4, type_from_remote_endpoint=UINT16, offset_from_remote_endpoint=0, nic_name=eth0, protocol=UDP, tcp_mode=Server, port=7200, remote_ip=255.255.255.255, exe_name=AsyncEthernet, swap_tx=off, swap_rx=off}
      mask prompts: ctrl_id "Controller ID"; nbr_to_remote_endpoint "Number of data to send"; type_to_remote_endpoint "Type of data to send"; offset_to_remote_endpoint "Byte offset of transmission buffer"; nbr_from_remote_endpoint "Number of data expected to be received"; type_from_remote_endpoint "Type of data expected to be received"; offset_from_remote_endpoint "Byte offset of reception buffer"; nic_name "Network interface name"; tcp_mode "TCP mode"; remote_ip "Remote IP address"; exe_name "Name of the executable"; swap_tx "Swap data endianness before transmission"; swap_rx "Swap data endianness after reception"
      mask help: Generic asynchronous process configuration block
      mask Help: eval('rtlab_help(''opasyncgenctrl'');');
      mask TypeOptions type_to_remote_endpoint: UINT8 | INT8 | UINT16 | INT16 | UINT32 | INT32 | FLOAT | DOUBLE
      mask TypeOptions type_from_remote_endpoint: UINT8 | INT8 | UINT16 | INT16 | UINT32 | INT32 | FLOAT | DOUBLE
      mask TypeOptions protocol: UDP | TCP
      mask TypeOptions tcp_mode: Client | Server
      mask Display: disp(sprintf('\nEthernet communication \ninterface controller\n'))
  B-width : SignalSpecification  Dimensions=nbr_from_remote_endpoint
  Constant : Constant  Value=1000
  Logo : opal_lib/Logo1  vide=[]
  Mux : Mux  Inputs=2
  OpAsyncRecv : rtlab/Communication/Asynchronous/OpAsyncRecv  ctl_id=ctrl_id  recv_id=ctrl_id  enable_param=off  fp1=1  fp2=2  fp3=3  fp4=4  fp5=5  sp1=string1  sp2=string2  sp3=string3  sp4=string4  sp5=string5
  OpAsyncSend : rtlab/Communication/Asynchronous/OpAsyncSend  ctl_id=ctrl_id  send_id=ctrl_id  mode=DONT_NEED_REPLY  enable_param=off  fp1=1  fp2=2  fp3=3  fp4=4  fp5=5  sp1=string1  sp2=string2  sp3=string3  sp4=string4  sp5=string5
  Terminator : Terminator
  Data received : Outport
  Status : Outport  Port=2
  wires:
  Data to send/1 -> OpAsyncSend/2
  Data trigger/1 -> OpAsyncSend/1
  OpAsyncSend/1 -> Mux/1
  OpAsyncRecv/1 -> Mux/2
  Mux/1 -> Status/1
  Constant/1 -> OpAsyncRecv/1
  OpAsyncRecv/2 -> Terminator/1
  OpAsyncRecv/3 -> B-width/1
  B-width/1 -> Data received/1

== system BANSHEE/SC_ctrl/Overall/currents/1ph_rms1 ==
  i : Inport
  Demux : Demux  Outputs=3
  o : Outport
  wires:
  Demux/1 -> o/1
  i/1 -> Demux/1

== system BANSHEE/SC_ctrl/Overall/currents/1ph_rms10 ==
  i : Inport
  Demux : Demux  Outputs=3
  o : Outport
  wires:
  Demux/1 -> o/1
  i/1 -> Demux/1

== system BANSHEE/SC_ctrl/Overall/currents/1ph_rms11 ==
  i : Inport
  Demux : Demux  Outputs=3
  o : Outport
  wires:
  Demux/1 -> o/1
  i/1 -> Demux/1

== system BANSHEE/SC_ctrl/Overall/currents/1ph_rms12 ==
  i : Inport
  Demux : Demux  Outputs=3
  o : Outport
  wires:
  Demux/1 -> o/1
  i/1 -> Demux/1

== system BANSHEE/SC_ctrl/Overall/currents/1ph_rms13 ==
  i : Inport
  Demux : Demux  Outputs=3
  o : Outport
  wires:
  Demux/1 -> o/1
  i/1 -> Demux/1

== system BANSHEE/SC_ctrl/Overall/currents/1ph_rms14 ==
  i : Inport
  Demux : Demux  Outputs=3
  o : Outport
  wires:
  Demux/1 -> o/1
  i/1 -> Demux/1

== system BANSHEE/SC_ctrl/Overall/currents/1ph_rms15 ==
  i : Inport
  Demux : Demux  Outputs=3
  o : Outport
  wires:
  Demux/1 -> o/1
  i/1 -> Demux/1

== system BANSHEE/SC_ctrl/Overall/currents/1ph_rms2 ==
  i : Inport
  Demux : Demux  Outputs=3
  o : Outport
  wires:
  Demux/1 -> o/1
  i/1 -> Demux/1

== system BANSHEE/SC_ctrl/Overall/currents/1ph_rms3 ==
  i : Inport
  Demux : Demux  Outputs=3
  o : Outport
  wires:
  Demux/1 -> o/1
  i/1 -> Demux/1

== system BANSHEE/SC_ctrl/Overall/currents/1ph_rms4 ==
  i : Inport
  Demux : Demux  Outputs=3
  o : Outport
  wires:
  Demux/1 -> o/1
  i/1 -> Demux/1

== system BANSHEE/SC_ctrl/Overall/currents/1ph_rms5 ==
  i : Inport
  Demux : Demux  Outputs=3
  o : Outport
  wires:
  Demux/1 -> o/1
  i/1 -> Demux/1

== system BANSHEE/SC_ctrl/Overall/currents/1ph_rms6 ==
  i : Inport
  Demux : Demux  Outputs=3
  o : Outport
  wires:
  Demux/1 -> o/1
  i/1 -> Demux/1

== system BANSHEE/SC_ctrl/Overall/currents/1ph_rms7 ==
  i : Inport
  Demux : Demux  Outputs=3
  o : Outport
  wires:
  Demux/1 -> o/1
  i/1 -> Demux/1

== system BANSHEE/SC_ctrl/Overall/currents/1ph_rms8 ==
  i : Inport
  Demux : Demux  Outputs=3
  o : Outport
  wires:
  Demux/1 -> o/1
  i/1 -> Demux/1

== system BANSHEE/SC_ctrl/Overall/currents/1ph_rms9 ==
  i : Inport
  Demux : Demux  Outputs=3
  o : Outport
  wires:
  Demux/1 -> o/1
  i/1 -> Demux/1

== system BANSHEE/SC_ctrl/Overall/currents/RMS_Calculator ==
  Signal : Inport
  Discrete  Mean value6 : powerlib_extras/Discrete Measurements/Discrete  Mean value  Freq=60  Vinit=0  Ts=Ts
  Product3 : Product  RndMeth=Zero
  Signed Sqrt : Sqrt  SaturateOnIntegerOverflow=on
  RMS_Signal : Outport
  wires:
  Signed Sqrt/1 -> RMS_Signal/1
  Discrete  Mean value6/1 -> Signed Sqrt/1
  Product3/1 -> Discrete  Mean value6/1
  Signal/1 -> Product3/2, Product3/1

== system BANSHEE/SC_ctrl/Overall/currents/RMS_Calculator1 ==
  Signal : Inport
  Discrete  Mean value6 : powerlib_extras/Discrete Measurements/Discrete  Mean value  Freq=60  Vinit=0  Ts=Ts
  Product3 : Product  RndMeth=Zero
  Signed Sqrt : Sqrt  SaturateOnIntegerOverflow=on
  RMS_Signal : Outport
  wires:
  Signed Sqrt/1 -> RMS_Signal/1
  Discrete  Mean value6/1 -> Signed Sqrt/1
  Product3/1 -> Discrete  Mean value6/1
  Signal/1 -> Product3/2, Product3/1

== system BANSHEE/SC_ctrl/Overall/currents/RMS_Calculator2 ==
  Signal : Inport
  Discrete  Mean value6 : powerlib_extras/Discrete Measurements/Discrete  Mean value  Freq=60  Vinit=0  Ts=Ts
  Product3 : Product  RndMeth=Zero
  Signed Sqrt : Sqrt  SaturateOnIntegerOverflow=on
  RMS_Signal : Outport
  wires:
  Signed Sqrt/1 -> RMS_Signal/1
  Discrete  Mean value6/1 -> Signed Sqrt/1
  Product3/1 -> Discrete  Mean value6/1
  Signal/1 -> Product3/2, Product3/1

== system BANSHEE/SM_UtilityService/HWCtrl_IOs/Woodward Outputs - Diesel - Gen2/DIO - Gr3 ==
  Dout : Inport
  Bus Creator : BusCreator  Inputs=1
  Bus Selector1 : BusSelector  OutputSignals=DI_CH08-15  OutputAsBus=on
  Conditioning1 : Subsystem
  DigitalIn1 : rtio_opalrt_common/DigitalIn  CtrlName='OpCtrl'  portNb=6  FcnNos=Slot 3 Module A Subsection 2  size=1  maxcount=8  count=8  sampleTime=0  numchan=8
      settings: AttributesFormatString=%<CtrlName>
  DigitalOut1 : rtio_opalrt_common/DigitalOut  CtrlName='OpCtrl'  portNb=6  FcnNos=Slot 3 Module B Subsection 2  size=1  maxcount=8  count=8  numchan=8
      settings: AttributesFormatString=%<CtrlName>
  Terminator1 : Terminator
  Terminator6 : Terminator
  DIn : Outport
  wires:
  DigitalOut1/1 -> Terminator1/1
  Dout/1 -> Bus Selector1/1
  Bus Selector1/1 -> DigitalOut1/1
  DigitalIn1/2 -> Terminator6/1
  DigitalIn1/1 -> Conditioning1/1(In1)  "DI_CH08-15"
  Bus Creator/1 -> DIn/1
  Conditioning1/1(Out1) -> Bus Creator/1

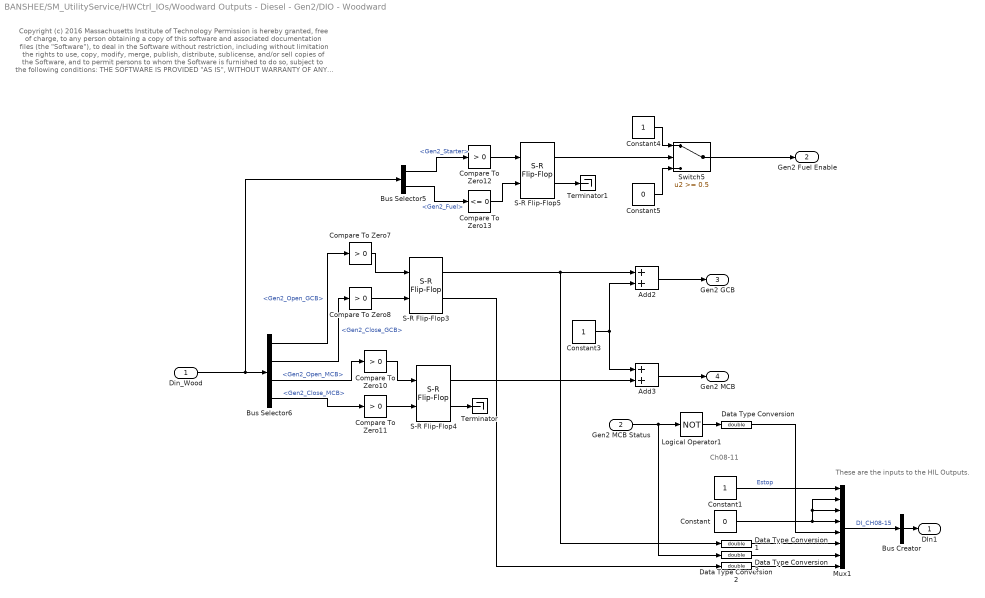
== system BANSHEE/SM_UtilityService/HWCtrl_IOs/Woodward Outputs - Diesel - Gen2/DIO - Woodward ==
  note: Copyright (c) 2016 Massachusetts Institute of Technology
      | Permission is hereby granted, free of charge, to any person obtaining a copy of this software and associated documentation files (the "Software"), to deal
      | in the Software without restriction, including without limitation the rights to use, copy, modify, merge, publish, distribute, sublicense, and/or sell copies of the
      | Software, and to permit persons to whom the Software is furnished to do so, subject to the following conditions:
      |
      | THE SOFTWARE IS PROVIDED "AS IS", WITHOUT WARRANTY OF ANY KIND, EXPRESS OR IMPLIED, INCLUDING BUT NOT LIMITED TO THE
      | WARRANTIES OF MERCHANTABILITY, FITNESS FOR A PARTICULAR PURPOSE AND NONINFRINGEMENT. IN NO EVENT SHALL THE AUTHORS
      | OR COPYRIGHT HOLDERS BE LIABLE FOR ANY CLAIM, DAMAGES OR OTHER LIABILITY, WHETHER IN AN ACTION OF CONTRACT, TORT OR
      | OTHERWISE, ARISING FROM, OUT OF OR IN CONNECTION WITH THE SOFTWARE OR THE USE OR OTHER DEALINGS IN THE SOFTWARE
  note: Ch08-11
  note: These are the inputs to
      | the HIL Outputs.
  Din_Wood : Inport
  Gen2 MCB Status : Inport  Port=2
  Add2 : Sum
  Add3 : Sum
  Bus Creator : BusCreator  Inputs=1
  Bus Selector5 : BusSelector  OutputSignals=DI_CH08-15.Gen2_Starter,DI_CH08-15.Gen2_Fuel
  Bus Selector6 : BusSelector  OutputSignals=DI_CH08-15.Gen2_Open_GCB,DI_CH08-15.Gen2_Close_GCB,DI_CH08-15.Gen2_Open_MCB,DI_CH08-15.Gen2_Close_MCB
  Compare To Zero{7..8,10..12} (5 alike) : simulink/Logic and Bit Operations/Compare To Zero  relop=>  OutDataTypeStr=boolean
  Compare To Zero13 : simulink/Logic and Bit Operations/Compare To Zero  relop=<=  OutDataTypeStr=boolean
  Constant : Constant  Value=0
  Constant1 : Constant
  Constant3 : Constant
  Constant4 : Constant
  Constant5 : Constant  Value=0
  Data Type Conversion{,1..3} (4 alike) : DataTypeConversion  OutDataTypeStr=double
  Logical Operator1 : Logic  Operator=NOT  AllPortsSameDT=off  OutDataTypeStr=boolean
  Mux1 : Mux  Inputs=8
  S-R Flip-Flop3 : simulink_extras/Flip Flops/S-R Flip-Flop  initial_condition=1
  S-R Flip-Flop4 : simulink_extras/Flip Flops/S-R Flip-Flop  initial_condition=1
  S-R Flip-Flop5 : simulink_extras/Flip Flops/S-R Flip-Flop  initial_condition=0
  Switch5 : Switch  Threshold=0.5
  Terminator : Terminator
  Terminator1 : Terminator
  DIn1 : Outport
  Gen2 Fuel Enable : Outport  Port=2
  Gen2 GCB : Outport  Port=3
  Gen2 MCB : Outport  Port=4
  wires:
  Constant1/1 -> Mux1/1  "Estop"
  Data Type Conversion3/1 -> Mux1/8
  Data Type Conversion2/1 -> Mux1/7
  Data Type Conversion1/1 -> Mux1/6
  Constant/1 -> Mux1/4, Mux1/3, Mux1/2
  S-R Flip-Flop5/2 -> Terminator1/1
  S-R Flip-Flop4/2 -> Terminator/1
  Din_Wood/1 -> Bus Selector5/1, Bus Selector6/1
  Bus Creator/1 -> DIn1/1
  Mux1/1 -> Bus Creator/1  "DI_CH08-15"
  S-R Flip-Flop3/1 -> Data Type Conversion1/1, Add2/1
  Bus Selector6/1 -> Compare To Zero7/1  "<Gen2_Open_GCB>"
  Compare To Zero7/1 -> S-R Flip-Flop3/1
  Compare To Zero8/1 -> S-R Flip-Flop3/2
  Bus Selector6/4 -> Compare To Zero11/1  "<Gen2_Close_MCB>"
  Compare To Zero11/1 -> S-R Flip-Flop4/2
  Bus Selector6/3 -> Compare To Zero10/1  "<Gen2_Open_MCB>"
  Compare To Zero10/1 -> S-R Flip-Flop4/1
  Bus Selector6/2 -> Compare To Zero8/1  "<Gen2_Close_GCB>"
  S-R Flip-Flop4/1 -> Add3/2
  Add2/1 -> Gen2 GCB/1
  Add3/1 -> Gen2 MCB/1
  Constant3/1 -> Add2/2, Add3/1
  Bus Selector5/1 -> Compare To Zero12/1  "<Gen2_Starter>"
  Bus Selector5/2 -> Compare To Zero13/1  "<Gen2_Fuel>"
  S-R Flip-Flop5/1 -> Switch5/2
  Compare To Zero12/1 -> S-R Flip-Flop5/1
  Constant5/1 -> Switch5/3
  Constant4/1 -> Switch5/1
  Compare To Zero13/1 -> S-R Flip-Flop5/2
  Switch5/1 -> Gen2 Fuel Enable/1
  Gen2 MCB Status/1 -> Logical Operator1/1, Data Type Conversion2/1
  S-R Flip-Flop3/2 -> Data Type Conversion3/1
  Logical Operator1/1 -> Data Type Conversion/1
  Data Type Conversion/1 -> Mux1/5

== system BANSHEE/SM_UtilityService/HWCtrl_IOs/Woodward Outputs - Diesel - Gen2/DOUT type config ==
  note: The Constants are used to select Digital Output type:
      | - 0: Time-Stamped Digital Output
      | - 1: Pulse-Width Modulated DIgital Output
  DataIn Send : rtio_opalrt_common/DataIn Send  CtrlName='OpCtrl'  FcnNos=11  width=1  portType=double  checkVersion=off  expectedId=0  expectedVersion=0  opComp=>=
      settings: AttributesFormatString=%<CtrlName>
  DataIn Send1 : rtio_opalrt_common/DataIn Send  CtrlName='OpCtrl'  FcnNos=12  width=1  portType=double  checkVersion=off  expectedId=0  expectedVersion=0  opComp=>=
      settings: AttributesFormatString=%<CtrlName>
  Subsection 3 DOUT type : Constant
  Subsection 4 DOUT type : Constant
  Terminator1 : Terminator
  Terminator2 : Terminator
  wires:
  Subsection 3 DOUT type/1 -> DataIn Send/1
  Subsection 4 DOUT type/1 -> DataIn Send1/1
  DataIn Send1/1 -> Terminator1/1
  DataIn Send/1 -> Terminator2/1
